simulink model "EKF"  (R2025b)
settings: Solver=FixedStepDiscrete  StartTime=0.0  StopTime=10.0  RelTol=1e-3
undefined symbols (not defined in the file): ekf_predict_dt, g_n, imu_sample_time, R_pos, R_vel, sigma_acc, sigma_ba, sigma_bg, sigma_gyr
libraries: simulink x1
settings Model: DataDictionary=StateEstDict.sldd  Creator=89447  LastModifiedBy=89447

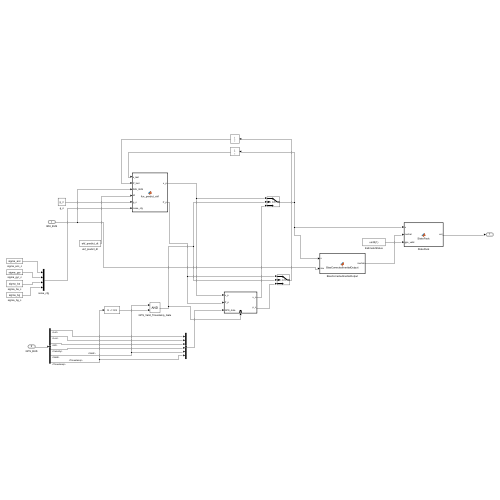
[thumbnail: Simulink's stored preview of the top-level diagram]
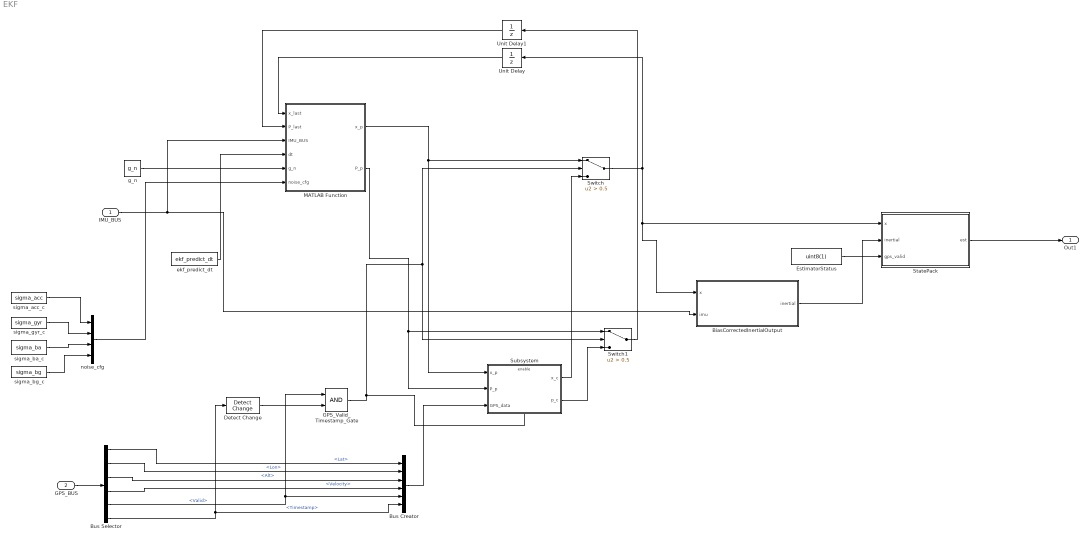
== system EKF ==
  IMU_BUS : Inport  OutDataTypeStr=Bus: IMU_BUS
  GPS_BUS : Inport  Port=2  OutDataTypeStr=Bus: GPS_BUS
  BiasCorrectedInertialOutput : MATLAB Function  TreatAsAtomicUnit=on
  Bus Creator : BusCreator  Inputs=6  OutDataTypeStr=Bus: GPS_BUS
  Bus Selector : BusSelector  OutputSignals=Lat,Lon,Alt,Velocity,Valid,Timestamp
  Detect Change : simulink/Logic and Bit Operations/Detect Change  vinit=0  OutDataTypeStr=boolean
  EstimatorStatus : Constant  Value=uint8(1)  OutDataTypeStr=uint8  SampleTime=imu_sample_time
  GPS_Valid_Timestamp_Gate : Logic  AllPortsSameDT=off  OutDataTypeStr=boolean
  MATLAB Function : MATLAB Function  TreatAsAtomicUnit=on
  StatePack : MATLAB Function  TreatAsAtomicUnit=on
  Subsystem : Subsystem
  Switch : Switch  Criteria=u2 > Threshold  Threshold=0.5  SaturateOnIntegerOverflow=off  InputSameDT=off
  Switch1 : Switch  Criteria=u2 > Threshold  Threshold=0.5  SaturateOnIntegerOverflow=off  InputSameDT=off
  Unit Delay : UnitDelay  SampleTime=-1  HasFrameUpgradeWarning=on
  Unit Delay1 : UnitDelay  SampleTime=-1  HasFrameUpgradeWarning=on
  ekf_predict_dt : Constant  Value=ekf_predict_dt  OutDataTypeStr=single
  g_n : Constant  Value=g_n  OutDataTypeStr=single
  noise_cfg : Mux
  sigma_acc_c : Constant  Value=sigma_acc  OutDataTypeStr=single
  sigma_ba_c : Constant  Value=sigma_ba  OutDataTypeStr=single
  sigma_bg_c : Constant  Value=sigma_bg  OutDataTypeStr=single
  sigma_gyr_c : Constant  Value=sigma_gyr  OutDataTypeStr=single
  Out1 : Outport  OutDataTypeStr=Bus: StateEstBus
  wires:
  MATLAB Function/1(x_p) -> Subsystem/1(x_p), Switch/1
  IMU_BUS/1 -> MATLAB Function/3(IMU_BUS), BiasCorrectedInertialOutput/2(imu)
  Bus Creator/1 -> Subsystem/3(GPS_data)
  Unit Delay/1 -> MATLAB Function/1(x_last)
  MATLAB Function/2(P_p) -> Subsystem/2(P_p), Switch1/1
  Switch/1 -> BiasCorrectedInertialOutput/1(x), StatePack/1(x), Unit Delay/1
  Subsystem/1(x_c) -> Switch/3
  Unit Delay1/1 -> MATLAB Function/2(P_last)
  Subsystem/2(p_c) -> Switch1/3
  Switch1/1 -> Unit Delay1/1
  GPS_BUS/1 -> Bus Selector/1
  sigma_acc_c/1 -> noise_cfg/1
  sigma_gyr_c/1 -> noise_cfg/2
  sigma_ba_c/1 -> noise_cfg/3
  sigma_bg_c/1 -> noise_cfg/4
  g_n/1 -> MATLAB Function/5(g_n)
  ekf_predict_dt/1 -> MATLAB Function/4(dt)
  noise_cfg/1 -> MATLAB Function/6(noise_cfg)
  EstimatorStatus/1 -> StatePack/3(gps_valid)
  StatePack/1(est) -> Out1/1
  Bus Selector/1 -> Bus Creator/1  "<Lat>"
  Bus Selector/2 -> Bus Creator/2  "<Lon>"
  Bus Selector/3 -> Bus Creator/3  "<Alt>"
  Bus Selector/4 -> Bus Creator/4  "<Velocity>"
  Bus Selector/5 -> Bus Creator/5, GPS_Valid_Timestamp_Gate/1  "<Valid>"
  Bus Selector/6 -> Bus Creator/6, Detect Change/1  "<Timestamp>"
  Detect Change/1 -> GPS_Valid_Timestamp_Gate/2
  GPS_Valid_Timestamp_Gate/1 -> Switch1/2, Switch/2, Subsystem/Enable
  BiasCorrectedInertialOutput/1(inertial) -> StatePack/2(inertial)

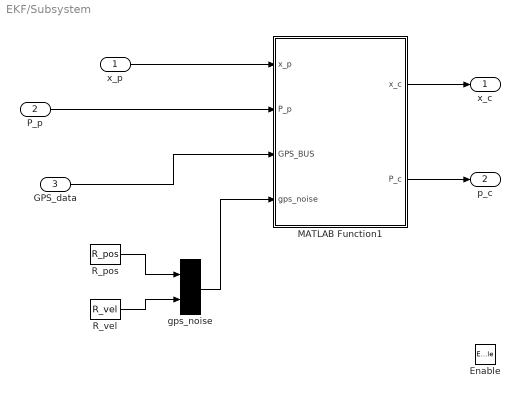
== system EKF/Subsystem ==
  x_p : Inport
  P_p : Inport  Port=2
  GPS_data : Inport  Port=3  OutDataTypeStr=Bus: GPS_BUS
  Enable : EnablePort
  MATLAB Function1 : MATLAB Function  TreatAsAtomicUnit=on
  R_pos : Constant  Value=R_pos  OutDataTypeStr=single
  R_vel : Constant  Value=R_vel  OutDataTypeStr=single
  gps_noise : Mux  Inputs=2
  x_c : Outport
  p_c : Outport  Port=2
  wires:
  MATLAB Function1/1(x_c) -> x_c/1
  GPS_data/1 -> MATLAB Function1/3(GPS_BUS)
  x_p/1 -> MATLAB Function1/1(x_p)
  P_p/1 -> MATLAB Function1/2(P_p)
  MATLAB Function1/2(P_c) -> p_c/1
  R_pos/1 -> gps_noise/1
  R_vel/1 -> gps_noise/2
  gps_noise/1 -> MATLAB Function1/4(gps_noise)

== matlab function EKF/BiasCorrectedInertialOutput ==
  data: x input; inertial output; imu input
function inertial = BiasCorrectedInertialOutput(x, imu)
%#codegen
gyro_bias = x(14:16);
accel_bias = x(11:13);
gyro_body = single(imu.Gyro - gyro_bias);
accel_body = single(imu.Accel - accel_bias);
inertial = single([gyro_body; accel_body]);
end

== matlab function EKF/StatePack ==
  data: x input; est output Bus: StateEstBus; inertial input; gps_valid input
function est = StatePack(x, inertial, gps_valid)
%#codegen
% x(16x1): [p;v;q;ba;bg]
% inertial(6x1): [bias-corrected gyro_body; bias-corrected accel_body]
est.Position_NED     = single(x(1:3));
est.Velocity_NED     = single(x(4:6));
est.Attitude_quat    = single(x(7:10));
est.AngularRate_Body = single(inertial(1:3));
est.Accel_Body       = single(inertial(4:6));
est.GyroBias         = single(x(14:16));
est.AccelBias        = single(x(11:13));
est.Wind_NED         = single([0;0;0]);
est.Status           = uint8(gps_valid);
end

== matlab function EKF/MATLAB Function ==
  data: x_last input single size=16; x_p output single size=16; P_last input single size=[15 15]; IMU_BUS input Bus: IMU_BUS; P_p output single size=[15 15]; dt input single size=1; g_n input single size=3; noise_cfg input single size=4
function [x_p, P_p] = fcn_predict_ekf(x_last, P_last, IMU_BUS, dt, g_n, noise_cfg)
% EKF 预测步
% 协方差在状态切空间 (15D) 上传播，通过线性化全状态运动学得到 Jacobian

sigma_acc = noise_cfg(1);
sigma_gyr = noise_cfg(2);
sigma_ba  = noise_cfg(3);
sigma_bg  = noise_cfg(4);

Q_c = diag([sigma_acc*ones(1,3), sigma_gyr*ones(1,3), sigma_ba*ones(1,3), sigma_bg*ones(1,3)]);

% --- 1. 状态提取与偏置补偿 ---
p = x_last(1:3); v = x_last(4:6); q = x_last(7:10);
ba = x_last(11:13); bg = x_last(14:16);

accel_corr = IMU_BUS.Accel - ba;
omega_corr = IMU_BUS.Gyro - bg;

% --- 2. 状态预测 (非线性动力学) ---
dq = quat_exp(omega_corr, dt);
q_p = quat_mult(q, dq);
q_p = quat_normalize(q_p);

C_bn = quat2rotm(q);
a_n = C_bn * accel_corr + g_n;
v_p = v + a_n * dt;
p_p = p + v * dt + 0.5 * a_n * dt^2;

x_p = [p_p; v_p; q_p; ba; bg];

% --- 3. 协方差预测 ---
% 连续时间状态转移 Jacobian (线性化全状态动力学)
F_c = zeros(15, 15);
a_sk = skew_sym(accel_corr);
w_sk = skew_sym(omega_corr);

F_c(1:3, 4:6)   = eye(3);
F_c(4:6, 7:9)   = -C_bn * a_sk;
F_c(4:6, 10:12) = -C_bn;
F_c(7:9, 7:9)   = -w_sk;
F_c(7:9, 13:15) = -eye(3);

F = eye(15) + F_c * dt;

G = zeros(15, 12);
G(4:6, 1:3)   = -C_bn;
G(7:9, 4:6)   = -eye(3);
G(10:12, 7:9) = eye(3);
G(13:15, 10:12)= eye(3);

Q_d = G * Q_c * G' * dt;
P_p = F * P_last * F' + Q_d;
P_p = (P_p + P_p') / 2;
end

== matlab function EKF/Subsystem/MATLAB Function1 ==
  data: x_p input single size=16; x_c output single size=16; P_p input single size=[15 15]; GPS_BUS input Bus: GPS_BUS; P_c output single size=[15 15]; gps_noise input single size=2
function [x_c, P_c] = fcn_update_ekf(x_p, P_p, GPS_BUS, gps_noise)
% EKF 更新步 — GPS 位置/速度观测
% 卡尔曼增益作用于状态切空间 (15D)，修正量通过流形上的 retraction 合入全状态
R_pos = gps_noise(1);
R_vel = gps_noise(2);

% --- 1. 观测向量 z (6x1) ---
z = [GPS_BUS.Lat; GPS_BUS.Lon; GPS_BUS.Alt; GPS_BUS.Velocity];

% --- 2. 观测 Jacobian H (6x15) ---
% 观测函数 h(x) = [p; v]，H = dh/dx 在切空间上的线性化
H = zeros(6, 15);
H(1:3, 1:3) = eye(3);
H(4:6, 4:6) = eye(3);

R = diag([R_pos*ones(1,3), R_vel*ones(1,3)]);

% --- 3. 卡尔曼增益 (15x6) ---
S = H * P_p * H' + R;
K = (P_p * H') / S;

% --- 4. 状态修正量 (15x1, 切空间) ---
innovation = z - [x_p(1:3); x_p(4:6)];
delta_x = K * innovation;

% --- 5. 修正量合入全状态 (流形 retraction) ---
x_c = x_p;
x_c(1:3)  = x_p(1:3)  + delta_x(1:3);
x_c(4:6)  = x_p(4:6)  + delta_x(4:6);
dq = quat_exp(delta_x(7:9), 1.0);
x_c(7:10) = quat_mult(dq, x_p(7:10));
x_c(7:10) = quat_normalize(x_c(7:10));
x_c(11:13) = x_p(11:13) + delta_x(10:12);
x_c(14:16) = x_p(14:16) + delta_x(13:15);

% --- 6. Joseph 形式协方差更新 ---
I = eye(15);
P_c = (I - K*H) * P_p * (I - K*H)' + K * R * K';
P_c = (P_c + P_c') / 2;
end
